simulink model "volt_simulink_block"  (R2019a)
settings: Solver=VariableStepAuto  StartTime=0.0  StopTime=5  RelTol=1e-3
settings Model: Creator=USER  LastModifiedBy=USER

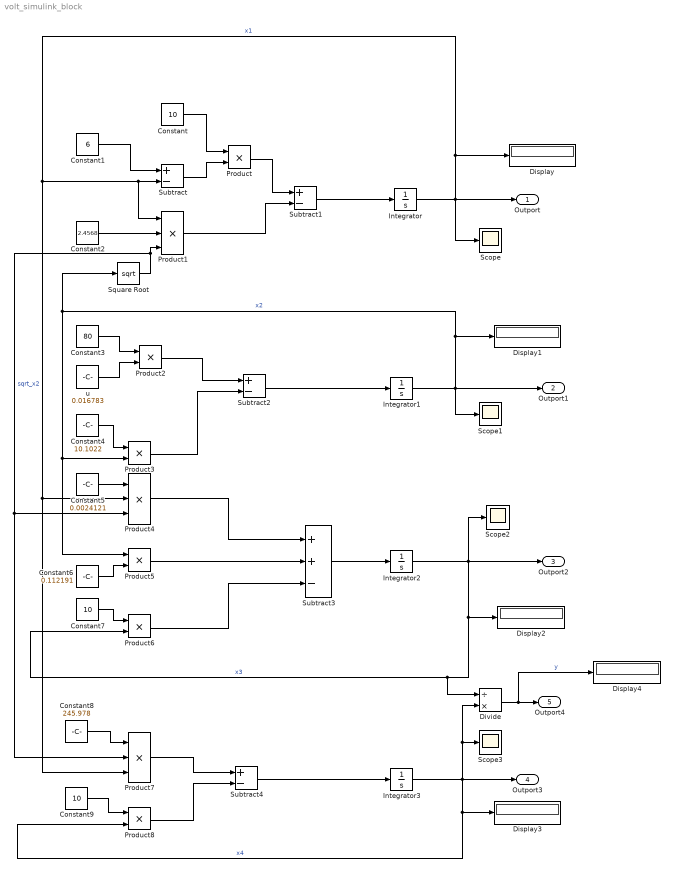
== system volt_simulink_block ==
  Constant : Constant  Value=10
  Constant1 : Constant  Value=6
  Constant2 : Constant  Value=2.4568
  Constant3 : Constant  Value=80
  Constant4 : Constant  Value=10.1022
  Constant5 : Constant  Value=0.0024121
  Constant6 : Constant  Value=0.112191
  Constant7 : Constant  Value=10
  Constant8 : Constant  Value=245.978
  Constant9 : Constant  Value=10
  Display{,1..4} (5 alike) : Display
  Divide : Product  Inputs=/*
  Integrator : Integrator  InitialCondition=6
  Integrator1 : Integrator  InitialCondition=8
  Integrator2 : Integrator
  Integrator3 : Integrator
  Product{,2..3,5..6,8} (6 alike) : Product
  Product1 : Product  Inputs=3
  Product4 : Product  Inputs=3
  Product7 : Product  Inputs=3
  Scope{,1..3} (4 alike) : Scope
  Square Root : Sqrt  SaturateOnIntegerOverflow=on
  Subtract{,1..2,4} (4 alike) : Sum  Inputs=+-
  Subtract3 : Sum  Inputs=++-
  u : Constant  Value=0.016783
  Outport : Outport
  Outport1 : Outport  Port=2
  Outport2 : Outport  Port=3
  Outport3 : Outport  Port=4
  Outport4 : Outport  Port=5
  wires:
  Constant1/1 -> Subtract/1
  Integrator/1 -> Scope/1, Subtract/2, Product1/1, Product7/3, Product4/2, Display/1, Outport/1  "x1"
  Constant/1 -> Product/1
  Subtract/1 -> Product/2
  Integrator1/1 -> Scope1/1, Square Root/1, Product5/1, Product3/2, Display1/1, Outport1/1  "x2"
  Square Root/1 -> Product4/3, Product7/2, Product1/3  "sqrt_x2"
  Constant2/1 -> Product1/2
  Product1/1 -> Subtract1/2
  Product/1 -> Subtract1/1
  Subtract1/1 -> Integrator/1
  Constant3/1 -> Product2/1
  u/1 -> Product2/2
  Product2/1 -> Subtract2/1
  Constant4/1 -> Product3/1
  Product3/1 -> Subtract2/2
  Subtract2/1 -> Integrator1/1
  Constant5/1 -> Product4/1
  Product4/1 -> Subtract3/1
  Constant6/1 -> Product5/2
  Product5/1 -> Subtract3/2
  Product6/1 -> Subtract3/3
  Subtract3/1 -> Integrator2/1
  Integrator2/1 -> Scope2/1, Display2/1, Divide/1, Product6/2, Outport2/1  "x3"
  Constant7/1 -> Product6/1
  Constant8/1 -> Product7/1
  Product7/1 -> Subtract4/1
  Constant9/1 -> Product8/1
  Product8/1 -> Subtract4/2
  Subtract4/1 -> Integrator3/1
  Integrator3/1 -> Divide/2, Scope3/1, Product8/2, Display3/1, Outport3/1  "x4"
  Divide/1 -> Display4/1, Outport4/1  "y"
